simulink model "Virtual_Exhaust_Aftertreatment_Controller_PRT"  (R2016b)
settings: Solver=FixedStepAuto  StartTime=0.0  StopTime=inf  FixedStep=VirtExhATCtrlr.tiSimnTiStep_C  RelTol=1e-3  SampleTimeConstraint=STIndependent  EnableMultiTasking=on
undefined symbols (not defined in the file or in its folder): CAL, SOUIT, T3LIMCL_COEOM_MSK_SY, T3LimCL_stMskEOM1_C, T3LimCL_stMskEOM2_C, T3LimCL_stMskEOM3_C, VirtExhATCtrlr_numHrznSize_CA
libraries: simulink x4
(part 2 of 5)

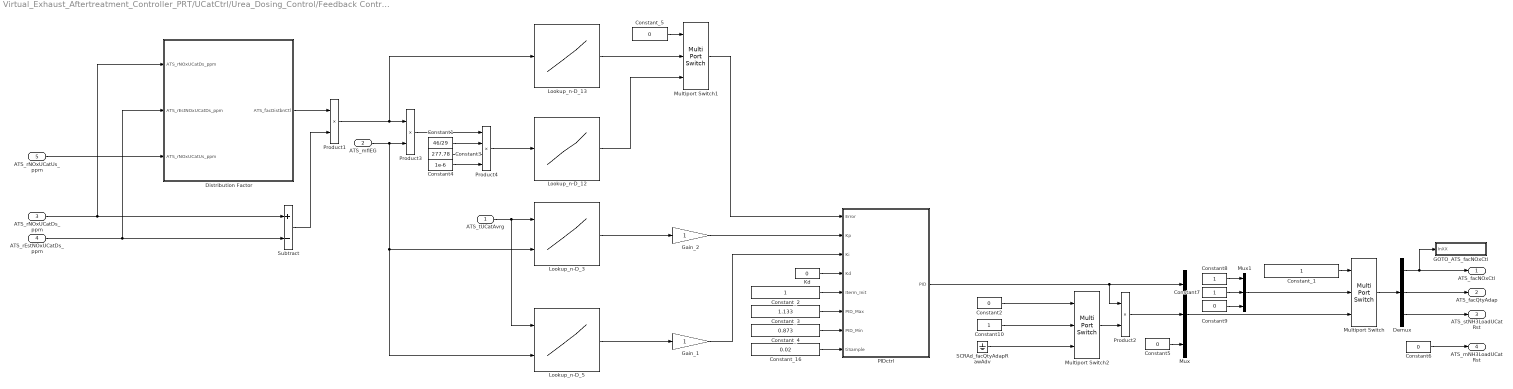
== system Virtual_Exhaust_Aftertreatment_Controller_PRT/UCatCtrl/Urea_Dosing_Control/Feedback Control ==
  "ATS_tUCatAvrg " : Inport
  ATS_mflEG : Inport  Port=2
  "ATS_rNOxUCatDs_ppm " : Inport  Port=3
  ATS_rEstNOxUCatDs_ppm : Inport  Port=4
  ATS_rNOxUCatUs_ppm : Inport  Port=5
  Constant1 : Constant  Value=46/29  SampleTime=-1
  Constant10 : Constant  SampleTime=-1
  Constant{2,5..6,9} (4 alike) : Constant  Value=0  SampleTime=-1
  Constant3 : Constant  Value=277.78  SampleTime=-1
  Constant4 : Constant  Value=1e-6  SampleTime=-1
  Constant7 : Constant  SampleTime=-1
  Constant8 : Constant  SampleTime=-1
  Constant_1 : Constant  SampleTime=-1
  Constant_16 : Constant  Value=0.02  SampleTime=-1
  Constant_2 : Constant  SampleTime=-1
  Constant_3 : Constant  Value=1.133  SampleTime=-1
  Constant_4 : Constant  Value=0.873  SampleTime=-1
  Constant_5 : Constant  Value=0  SampleTime=-1
  Demux : Demux  Outputs=3
  Distribution Factor : Subsystem
  GOTO_ATS_facNOxCtl : Subsystem  mask{SIG='ATS_facNOxCtl'}
      mask prompts: SIG "Log Signal Name"
      mask init: same as Virtual_Exhaust_Aftertreatment_Controller_PRT/UCatCtrl/SCR_Prediction/GOTO_ATS_etaEstNOxCnvUCat
      mask Display: fprintf(SIG);
  Gain_1 : Gain
  Gain_2 : Gain
  Kd : Constant  Value=0  SampleTime=-1
  Lookup_n-D_12 : Lookup_n-D  NumberOfTableDimensions=1  BreakpointsForDimension1=[0;10;20;30;40;50;55;60]  BreakpointsForDimension2=[159.96 449.96]  Table=[1;1;1;1;1;1;1;1]  ExtrapMethod=Clip  UseLastTableValue=on  RndMeth=Simplest  InputSameDT=on
  Lookup_n-D_13 : Lookup_n-D  NumberOfTableDimensions=1  BreakpointsForDimension1=[-500;-300;-50;0;50;100;150;175]  BreakpointsForDimension2=[159.96 449.96]  Table=[-1;-0.5;-0.14;0;0.15;0.4;0.8;1]  ExtrapMethod=Clip  UseLastTableValue=on  RndMeth=Simplest  InputSameDT=on
  Lookup_n-D_3 : Lookup_n-D  BreakpointsForDimension1=[0;200;400;600;800;1000;1200;1400]  BreakpointsForDimension2=[149.96 199.96 249.96 299.96 349.96 399.96 449.96 499.96]  Table=[0.15 0.15 0.15 0.15 0.12 0.09 0.06 0.03;0.136 0.136 0.136 0.136 0.109 0.081 0.054 0.027;0.121 0.121 0.121 0.121 0.097 0.073 0.049 0.024;0.107 0.107 0.107 0.107 0.086 0.064 0.043 0.021;0.093 0.093 0.093 0.093 0.074 0.056 0.037 0.019;0.079 0.079 0.079 0.079 0.063 0.047 0.031 0.016;0.064 0.064 0.064 0.064 0.051 0.039 0.026 0.013;0.05 0.05 0.05 0.05 0.04 0.03 0.02 0.01]  ExtrapMethod=Clip  UseLastTableValue=on  RndMeth=Simplest  InputSameDT=on
  Lookup_n-D_5 : Lookup_n-D  BreakpointsForDimension1=[0;200;400;600;800;1000;1200;1400]  BreakpointsForDimension2=[249.96 299.96 324.96 349.96 374.96 399.96 424.96 449.96]  Table=[0.1 0.068 0.052 0.036 0.02 0.0167 0.0133 0.01;0.1 0.068 0.052 0.036 0.02 0.0167 0.0133 0.01;0.1 0.068 0.052 0.036 0.02 0.0167 0.0133 0.01;0.1 0.068 0.052 0.036 0.02 0.0167 0.0133 0.01;0.1 0.068 0.052 0.036 0.02 0.0167 0.0133 0.01;0.1 0.068 0.052 0.036 0.02 0.0167 0.0133 0.01;0.1 0.068 0.052 0.036 0.02 0.0167 0.0133 0.01;0.1 0.068 0.052 0.036 0.02 0.0167 0.0133 0.01]  ExtrapMethod=Clip  UseLastTableValue=on  RndMeth=Simplest  InputSameDT=on
  Multiport Switch : MultiPortSwitch  DataPortOrder=Zero-based contiguous  Inputs=2
  Multiport Switch1 : MultiPortSwitch  DataPortOrder=Zero-based contiguous  Inputs=2
  Multiport Switch2 : MultiPortSwitch  DataPortOrder=Zero-based contiguous  Inputs=2
  Mux : Mux  Inputs=3
  Mux1 : Mux  Inputs=3
  PIDctrl : Subsystem
  Product1 : Product  RndMeth=Zero
  Product2 : Product  RndMeth=Zero
  Product3 : Product  RndMeth=Zero
  Product4 : Product  Inputs=4  RndMeth=Zero
  SCRAd_facQtyAdapRawAdv : Ground
  Subtract : Sum  Inputs=+-
  ATS_facNOxCtl : Outport
  ATS_facQtyAdap : Outport  Port=2
  ATS_stNH3LoadUCatRst : Outport  Port=3
  ATS_mNH3LoadUCatRst : Outport  Port=4
  wires:
  "ATS_tUCatAvrg "/1 -> Lookup_n-D_5/1, Lookup_n-D_3/1
  Lookup_n-D_5/1 -> Gain_1/1
  ATS_mflEG/1 -> Lookup_n-D_5/2, Lookup_n-D_3/2, Product3/2
  Lookup_n-D_3/1 -> Gain_2/1
  "ATS_rNOxUCatDs_ppm "/1 -> Distribution Factor/1("ATS_rNOxUCatDs_ppm "), Subtract/1
  PIDctrl/1(PID) -> Product2/1, Mux/1
  Subtract/1 -> Product1/2
  Demux/2 -> ATS_facQtyAdap/1
  Multiport Switch2/1 -> Product2/2
  ATS_rEstNOxUCatDs_ppm/1 -> Distribution Factor/2(ATS_rEstNOxUCatDs_ppm), Subtract/2
  ATS_rNOxUCatUs_ppm/1 -> Distribution Factor/3(ATS_rNOxUCatUs_ppm)
  Distribution Factor/1(ATS_facDistbnCtl) -> Product1/1
  Product1/1 -> Lookup_n-D_13/1, Product3/1
  Lookup_n-D_13/1 -> Multiport Switch1/2
  Product3/1 -> Product4/1
  Constant1/1 -> Product4/2
  Constant3/1 -> Product4/3
  Constant4/1 -> Product4/4
  Product4/1 -> Lookup_n-D_12/1
  Constant_5/1 -> Multiport Switch1/1
  Lookup_n-D_12/1 -> Multiport Switch1/3
  Multiport Switch1/1 -> PIDctrl/1(Error)
  Gain_1/1 -> PIDctrl/3(Ki)
  Gain_2/1 -> PIDctrl/2(Kp)
  Constant2/1 -> Multiport Switch2/1
  Constant10/1 -> Multiport Switch2/2
  SCRAd_facQtyAdapRawAdv/1 -> Multiport Switch2/3
  Constant6/1 -> ATS_mNH3LoadUCatRst/1
  Demux/3 -> ATS_stNH3LoadUCatRst/1
  Mux/1 -> Multiport Switch/3
  Constant_1/1 -> Multiport Switch/1
  Mux1/1 -> Multiport Switch/2
  Product2/1 -> Mux/2
  Constant5/1 -> Mux/3
  Constant8/1 -> Mux1/1
  Constant9/1 -> Mux1/3
  Multiport Switch/1 -> Demux/1
  Demux/1 -> ATS_facNOxCtl/1, GOTO_ATS_facNOxCtl/1(InXX)
  Constant_16/1 -> PIDctrl/8(tiSample)
  Kd/1 -> PIDctrl/4(Kd)
  Constant_2/1 -> PIDctrl/5(Iterm_Init)
  Constant_4/1 -> PIDctrl/7(PID_Min)
  Constant7/1 -> Mux1/2
  Constant_3/1 -> PIDctrl/6(PID_Max)

== system Virtual_Exhaust_Aftertreatment_Controller_PRT/UCatCtrl/Urea_Dosing_Control/GOTO_ATS_facQtyAdap ==
  InXX : Inport
  GainXX : Subsystem
  tag scope: ATS_facQtyAdap=global
  wires:
  InXX/1 -> GainXX/1(In)
  GainXX/1(Out) -> [ATS_facQtyAdap]  "ATS_facQtyAdap"

== system Virtual_Exhaust_Aftertreatment_Controller_PRT/UCatCtrl/Urea_Dosing_Control/GOTO_ATS_mNH3LdNom ==
  InXX : Inport
  GainXX : Subsystem
  tag scope: ATS_mNH3LdNom=global
  wires:
  GainXX/1(Out) -> [ATS_mNH3LdNom]  "ATS_mNH3LdNom"
  InXX/1 -> GainXX/1(In)

== system Virtual_Exhaust_Aftertreatment_Controller_PRT/UCatCtrl/Urea_Dosing_Control/GOTO_ATS_mNH3LoadUCatRst ==
  InXX : Inport
  GainXX : Subsystem
  tag scope: ATS_mNH3LoadUCatRst=global
  wires:
  InXX/1 -> GainXX/1(In)
  GainXX/1(Out) -> [ATS_mNH3LoadUCatRst]  "ATS_mNH3LoadUCatRst"

== system Virtual_Exhaust_Aftertreatment_Controller_PRT/UCatCtrl/Urea_Dosing_Control/GOTO_ATS_mflNH3Cnv_mgps ==
  InXX : Inport
  GainXX : Subsystem
  tag scope: ATS_mflNH3Cnv_mgps=global
  wires:
  InXX/1 -> GainXX/1(In)
  GainXX/1(Out) -> [ATS_mflNH3Cnv_mgps]  "ATS_mflNH3Cnv_mgps"

== system Virtual_Exhaust_Aftertreatment_Controller_PRT/UCatCtrl/Urea_Dosing_Control/GOTO_ATS_mflNH3CurrEfc_mgps ==
  InXX : Inport
  GainXX : Subsystem
  tag scope: ATS_mflNH3CurrEfc_mgps=global
  wires:
  InXX/1 -> GainXX/1(In)
  GainXX/1(Out) -> [ATS_mflNH3CurrEfc_mgps]  "ATS_mflNH3CurrEfc_mgps"

== system Virtual_Exhaust_Aftertreatment_Controller_PRT/UCatCtrl/Urea_Dosing_Control/GOTO_ATS_mflNH3DpstLmt_mgps ==
  InXX : Inport
  GainXX : Subsystem
  tag scope: ATS_mflNH3DpstLmt_mgps=global
  wires:
  GainXX/1(Out) -> [ATS_mflNH3DpstLmt_mgps]  "ATS_mflNH3DpstLmt_mgps"
  InXX/1 -> GainXX/1(In)

== system Virtual_Exhaust_Aftertreatment_Controller_PRT/UCatCtrl/Urea_Dosing_Control/GOTO_ATS_mflNH3MetAdapDes_mgps ==
  InXX : Inport
  GainXX : Subsystem
  tag scope: ATS_mflNH3MetAdapDes_mgps=global
  wires:
  GainXX/1(Out) -> [ATS_mflNH3MetAdapDes_mgps]  "ATS_mflNH3MetAdapDes_mgps"
  InXX/1 -> GainXX/1(In)

== system Virtual_Exhaust_Aftertreatment_Controller_PRT/UCatCtrl/Urea_Dosing_Control/GOTO_ATS_mflNH3PreCtl_mgps ==
  InXX : Inport
  GainXX : Subsystem
  tag scope: ATS_mflNH3PreCtl_mgps=global
  wires:
  InXX/1 -> GainXX/1(In)
  GainXX/1(Out) -> [ATS_mflNH3PreCtl_mgps]  "ATS_mflNH3PreCtl_mgps"

== system Virtual_Exhaust_Aftertreatment_Controller_PRT/UCatCtrl/Urea_Dosing_Control/GOTO_ATS_mflNH3_mgps ==
  InXX : Inport
  GainXX : Subsystem
  tag scope: ATS_mflNH3_mgps=global
  wires:
  InXX/1 -> GainXX/1(In)
  GainXX/1(Out) -> [ATS_mflNH3_mgps]  "ATS_mflNH3_mgps"

== system Virtual_Exhaust_Aftertreatment_Controller_PRT/UCatCtrl/Urea_Dosing_Control/GOTO_ATS_mflNOxUs_mgps ==
  InXX : Inport
  GainXX : Subsystem
  tag scope: ATS_mflNOxUs_mgps=global
  wires:
  GainXX/1(Out) -> [ATS_mflNOxUs_mgps]  "ATS_mflNOxUs_mgps"
  InXX/1 -> GainXX/1(In)

== system Virtual_Exhaust_Aftertreatment_Controller_PRT/UCatCtrl/Urea_Dosing_Control/GOTO_ATS_stNH3LoadUCatRst ==
  InXX : Inport
  GainXX : Subsystem
  tag scope: ATS_stNH3LoadUCatRst=global
  wires:
  GainXX/1(Out) -> [ATS_stNH3LoadUCatRst]  "ATS_stNH3LoadUCatRst"
  InXX/1 -> GainXX/1(In)

== system Virtual_Exhaust_Aftertreatment_Controller_PRT/UCatCtrl/Urea_Dosing_Control/GOTO_ATS_stUDosing ==
  InXX : Inport
  GainXX : Subsystem
  tag scope: ATS_stUDosing=global
  wires:
  InXX/1 -> GainXX/1(In)
  GainXX/1(Out) -> [ATS_stUDosing]  "ATS_stUDosing"

== system Virtual_Exhaust_Aftertreatment_Controller_PRT/UCatCtrl/Urea_Dosing_Control/GOTO_EvpMod_tUCatUsT ==
  InXX : Inport
  GainXX : Subsystem
  tag scope: EvpMod_tUCatUsT=global
  wires:
  InXX/1 -> GainXX/1(In)
  GainXX/1(Out) -> [EvpMod_tUCatUsT]  "EvpMod_tUCatUsT"

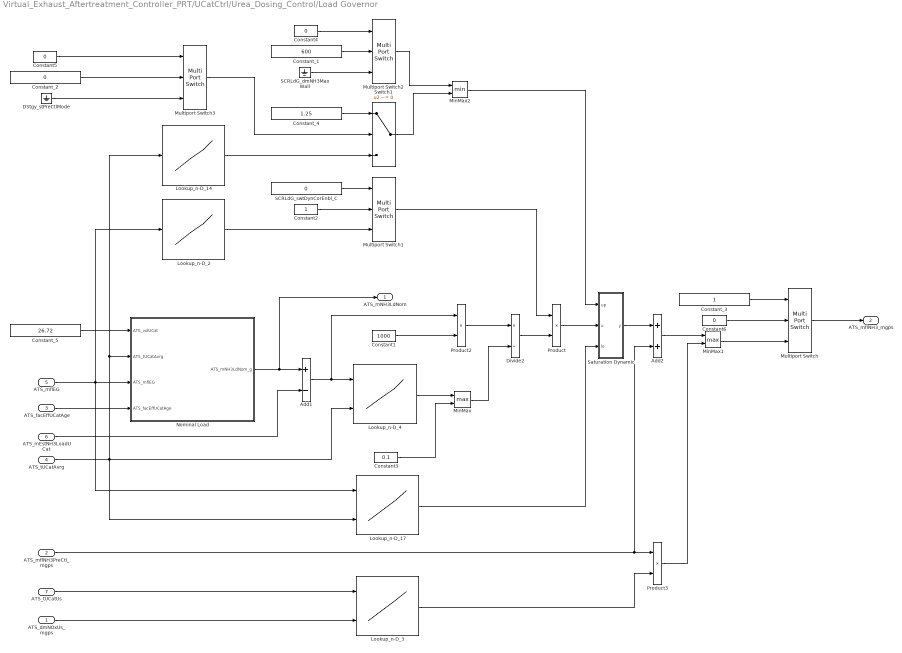
== system Virtual_Exhaust_Aftertreatment_Controller_PRT/UCatCtrl/Urea_Dosing_Control/Load Governor ==
  ATS_dmNOxUs_mgps : Inport
  ATS_mflNH3PreCtl_mgps : Inport  Port=2
  ATS_facEffUCatAge : Inport  Port=3
  ATS_tUCatAvrg : Inport  Port=4
  ATS_mflEG : Inport  Port=5
  ATS_mEstNH3LoadUCat : Inport  Port=6
  ATS_tUCatUs : Inport  Port=7
  Add1 : Sum  Inputs=+-
  Add2 : Sum
  Constant1 : Constant  Value=1000  SampleTime=-1
  Constant2 : Constant  SampleTime=-1
  Constant3 : Constant  Value=0.1  SampleTime=-1
  Constant4 : Constant  Value=0  SampleTime=-1
  Constant5 : Constant  Value=0  SampleTime=-1
  Constant6 : Constant  Value=0  SampleTime=-1
  Constant_1 : Constant  Value=600  SampleTime=-1
  Constant_2 : Constant  Value=0  SampleTime=-1
  Constant_3 : Constant  SampleTime=-1
  Constant_4 : Constant  Value=1.25  SampleTime=-1
  Constant_5 : Constant  Value=26.72  SampleTime=-1
  DStgy_stPreCtlMode : Ground
  Divide2 : Product  Inputs=*/
  Lookup_n-D_14 : Lookup_n-D  NumberOfTableDimensions=1  BreakpointsForDimension1=[159.96;229.96;299.96;369.96;439.96;509.96;579.96;649.96]  BreakpointsForDimension2=[159.96 449.96]  Table=[365;365;365;365;365;365;365;365]  ExtrapMethod=Clip  UseLastTableValue=on  RndMeth=Simplest  InputSameDT=on
  Lookup_n-D_17 : Lookup_n-D  BreakpointsForDimension1=[100;300;500;700;900;1100;1300;1500;1700;1900]  BreakpointsForDimension2=[159.96 449.96]  Table=[-50 -70;-55 -80;-65 -90;-75 -100;-90 -120;-105 -150;-130 -180;-160 -220;-195 -290;-250 -365]  ExtrapMethod=Clip  UseLastTableValue=on  RndMeth=Simplest  InputSameDT=on
  Lookup_n-D_2 : Lookup_n-D  NumberOfTableDimensions=1  BreakpointsForDimension1=[150;250;350;500;700;1000;1250;1500]  BreakpointsForDimension2=[159.96 449.96]  Table=[1;1;1;1;1;0.98;0.95;0.92]  ExtrapMethod=Clip  UseLastTableValue=on  RndMeth=Simplest  InputSameDT=on
  Lookup_n-D_3 : Lookup_n-D  BreakpointsForDimension1=[99.96;199.96;299.96;399.96;499.96;599.96]  BreakpointsForDimension2=[0 100 200 300 400 500]  Table=[0.5 0.5 0.5 0.5 0.5 0.5;0.5 0.5 0.5 0.5 0.5 0.5;0.5 0.5 0.5 0.5 0.5 0.5;0.5 0.5 0.5 0.5 0.5 0.5;0.5 0.5 0.5 0.5 0.5 0.5;0.5 0.5 0.5 0.5 0.5 0.5]  ExtrapMethod=Clip  UseLastTableValue=on  RndMeth=Simplest  InputSameDT=on
  Lookup_n-D_4 : Lookup_n-D  BreakpointsForDimension1=[-10;-5;-3;-2;-1;0.025000000372529;1;2;3;5;10]  BreakpointsForDimension2=[159.96 449.96]  Table=[27.5 27.5;43 35;57 45;65 60;74 74;70 0.1;35 2.8;25 5.5;22 8.3;22 13.8;27.5 27.5]  ExtrapMethod=Clip  UseLastTableValue=on  RndMeth=Simplest  InputSameDT=on
  MinMax : MinMax  Function=max  Inputs=2
  MinMax1 : MinMax  Function=max  Inputs=2
  MinMax2 : MinMax  Inputs=2
  Multiport Switch{,1..3} (4 alike) : MultiPortSwitch  DataPortOrder=Zero-based contiguous  Inputs=2
  Nominal Load : Subsystem
  Product : Product
  Product2 : Product  RndMeth=Zero
  Product3 : Product
  SCRLdG_dmNH3MaxWall : Ground
  SCRLdG_swtDynCorEnbl_C : Constant  Value=0  SampleTime=-1
  Saturation Dynamic : Subsystem  mask(Saturation Dynamic){OutMin=[], OutMax=[], OutDataTypeStr=Inherit: Same as second input, OutputDataTypeScalingMode=Same as second input, OutDataType=fixdt(1, 16), OutScaling=2^-10, LockScale=off, RndMeth=Floor, DoSatur=off}
      mask prompts: OutMin "Simulink:masks:OutputMinimum_MP"; OutMax "Simulink:masks:OutputMaximum_MP"; OutDataTypeStr "Simulink:masks:OutputDataType_MP"; OutputDataTypeScalingMode "Simulink:masks:OutputDataTypeMode_MP"; OutDataType "Simulink:masks:OutputDataTypeegFixdt116Fixdtsingle_MP"; OutScaling "Simulink:masks:OutputScalingSlopeEg29OrSlopeBias_MP"; LockScale "Simulink:masks:LockOutputDataTypeAgainstFxpTools_MP"; RndMeth "Simulink:masks:IntegerRoundingMode_MP"; DoSatur "Simulink:masks:SaturateOnIntegerOverflow_MP"
      mask help: Simulink:masks:SaturationDynamic_MD
      mask init: same as Virtual_Exhaust_Aftertreatment_Controller_PRT/UCatCtrl/Urea_Dosing_Control/Saturation Dynamic
      mask Callback OutDataTypeStr: fixptdialog(gcbh)
      mask TypeOptions OutputDataTypeScalingMode: double | single | int8 | uint8 | int16 | uint16 | int32 | uint32 | Specify via dialog | Same as second input
      mask Callback OutputDataTypeScalingMode: fixptdialog(gcbh)
      mask Callback OutDataType: fixptdialog(gcbh)
      mask TypeOptions RndMeth: Simulink:masks:Ceiling | Simulink:masks:Convergent | Simulink:masks:Floor | Simulink:masks:Nearest | Simulink:masks:Round | Simulink:masks:Simplest | Simulink:masks:Zero
      mask Display: plot([0.15 0.85],[.5 .5],[.5 .5],[0.05 0.95],0.15+0.7*[0 .25 .75 1],0.05+0.9*[.25 .25 .75 .75]);
  Switch1 : Switch  Criteria=u2 ~= 0  Threshold=SOUIT
  ATS_mNH3LdNom : Outport
  ATS_mflNH3_mgps : Outport  Port=2
  wires:
  Nominal Load/1(ATS_mNH3LdNom_g) -> ATS_mNH3LdNom/1, Add1/1
  ATS_mEstNH3LoadUCat/1 -> Add1/2
  Add1/1 -> Lookup_n-D_4/1, Product2/1
  ATS_tUCatAvrg/1 -> Nominal Load/2(ATS_tUCatAvrg), Lookup_n-D_14/1, Lookup_n-D_17/2, Lookup_n-D_4/2
  Lookup_n-D_4/1 -> MinMax/1
  Constant3/1 -> MinMax/2
  Constant1/1 -> Product2/2
  Product2/1 -> Divide2/1
  MinMax/1 -> Divide2/2
  ATS_mflNH3PreCtl_mgps/1 -> Add2/2, Product3/1
  MinMax1/1 -> Multiport Switch/3
  ATS_facEffUCatAge/1 -> Nominal Load/4(ATS_facEffUCatAge)
  Constant_5/1 -> Nominal Load/1(ATS_volUCat)
  Lookup_n-D_17/1 -> Saturation Dynamic/3(lo)
  Saturation Dynamic/1(y) -> Add2/1
  Product/1 -> Saturation Dynamic/2(u)
  Lookup_n-D_2/1 -> Multiport Switch1/3
  ATS_mflEG/1 -> Lookup_n-D_2/1, Lookup_n-D_17/1, Nominal Load/3(ATS_mflEG)
  Lookup_n-D_3/1 -> Product3/2
  Product3/1 -> MinMax1/2
  Divide2/1 -> Product/2
  Add2/1 -> MinMax1/1
  SCRLdG_swtDynCorEnbl_C/1 -> Multiport Switch1/1
  Constant2/1 -> Multiport Switch1/2
  Multiport Switch1/1 -> Product/1
  Lookup_n-D_14/1 -> Switch1/3
  Switch1/1 -> MinMax2/2
  Multiport Switch2/1 -> MinMax2/1
  MinMax2/1 -> Saturation Dynamic/1(up)
  ATS_tUCatUs/1 -> Lookup_n-D_3/1
  ATS_dmNOxUs_mgps/1 -> Lookup_n-D_3/2
  SCRLdG_dmNH3MaxWall/1 -> Multiport Switch2/3
  Constant4/1 -> Multiport Switch2/1
  Constant_1/1 -> Multiport Switch2/2
  Constant_4/1 -> Switch1/1
  Constant5/1 -> Multiport Switch3/1
  DStgy_stPreCtlMode/1 -> Multiport Switch3/3
  Constant_2/1 -> Multiport Switch3/2
  Multiport Switch3/1 -> Switch1/2
  Constant_3/1 -> Multiport Switch/1
  Constant6/1 -> Multiport Switch/2
  Multiport Switch/1 -> ATS_mflNH3_mgps/1

== system Virtual_Exhaust_Aftertreatment_Controller_PRT/UCatCtrl/Urea_Dosing_Control/SCRMod Wall Film ==
  ATS_mflNH3Cnv_mgps : Inport
  Constant_1 : Constant  Value=0  SampleTime=-1
  Multiport Switch1 : MultiPortSwitch  DataPortOrder=Zero-based contiguous  Inputs=2
  SCRMod_dmNH3CurrEff : Ground
  ATS_mflNH3CurrEfc_mgps : Outport
  wires:
  SCRMod_dmNH3CurrEff/1 -> Multiport Switch1/3
  Constant_1/1 -> Multiport Switch1/1
  Multiport Switch1/1 -> ATS_mflNH3CurrEfc_mgps/1
  ATS_mflNH3Cnv_mgps/1 -> Multiport Switch1/2

== system Virtual_Exhaust_Aftertreatment_Controller_PRT/UCatCtrl/Urea_Dosing_Control/Saturation Dynamic ==
  up : Inport
  u : Inport  Port=2
  lo : Inport  Port=3
  Data Type Duplicate : DataTypeDuplicate  DisableCoverage=on
  Data Type Propagation : S-Function  FunctionName=sfix_dtprop  Parameters=14,PropDataTypeMode,(getdatatypespecs(PropDataType,PropScaling,DblOver,0, 0, PropDataTypeMode, PropScalingMode)),IfRefDouble,IfRefSingle,IsSigned,NumBitsBase,NumBitsMult,NumBitsAdd,(sort(reshape(round(NumBitsAllowFinal), prod(size(NumBitsAllowFinal)),1))),PropScalingMode,ValuesUsedBestPrec,SlopeBase,SlopeMult,SlopeAdd,BiasBase,BiasMult,BiasAdd,DblOver  SFunctionDeploymentMode=off  EnableBusSupport=off  mask(Data Type Propagation){PropDataTypeMode=Inherit via propagation rule, PropDataType=fixdt(1, 16), IfRefDouble=double, IfRefSingle=single, IsSigned=IsSigned1, NumBitsBase=NumBits1, NumBitsMult=1, NumBitsAdd=0, NumBitsAllowFinal=1:128, PropScalingMode=Inherit via propagation rule, PropScaling=2^-10, ValuesUsedBestPrec=[5 -7], SlopeBase=Slope1, SlopeMult=1, SlopeAdd=0, BiasBase=Bias1, BiasMult=1, BiasAdd=0}
      mask prompts: PropDataTypeMode "Simulink:masks:x1PropagatedDataType_MP"; PropDataType "Simulink:masks:x11PropagatedDataTypeegFixdt116Fixdtsingle_MP"; IfRefDouble "Simulink:masks:x11IfAnyReferenceInputIsDoubleOutputIs_MP"; IfRefSingle "Simulink:masks:x12IfAnyReferenceInputIsSingleOutputIs_MP"; IsSigned "Simulink:masks:x13IsSigned_MP"; NumBitsBase "Simulink:masks:x141NumberofBitsBase_MP"; NumBitsMult "Simulink:masks:x142NumberofBitsMultiplicativeAdjustment_MP"; NumBitsAdd "Simulink:masks:x143NumberofBitsAdditiveAdjustment_MP"; NumBitsAllowFinal "Simulink:masks:x144NumberofBitsAllowableFinalValues_MP"; PropScalingMode "Simulink:masks:x2PropagatedScaling_MP"; PropScaling "Simulink:masks:x21PropagatedScalingSlopeEg29OrSlopeBiasEg1253_MP"; ValuesUsedBestPrec "Simulink:masks:x21ValuesUsedToDetermineBestPrecisionScaling_MP"; SlopeBase "Simulink:masks:x211SlopeBase_MP"; SlopeMult "Simulink:masks:x212SlopeMultiplicativeAdjustment_MP"; SlopeAdd "Simulink:masks:x213SlopeAdditiveAdjustment_MP"; BiasBase "Simulink:masks:x221BiasBase_MP"; BiasMult "Simulink:masks:x222BiasMultiplicativeAdjustment_MP"; BiasAdd "Simulink:masks:x223BiasAdditiveAdjustment_MP"
      mask help: Simulink:masks:DataTypePropagation_MD
      mask init:
      | DblOver = 0;
      mask TypeOptions PropDataTypeMode: Simulink:masks:SpecifyViaDialog | Simulink:masks:InheritViaPropagationRule
      mask Callback PropDataTypeMode: fixptdialog(gcbh)
      mask Callback PropDataType: fixptdialog(gcbh)
      mask TypeOptions IfRefDouble: Simulink:masks:double | Simulink:masks:single
      mask TypeOptions IfRefSingle: Simulink:masks:double | Simulink:masks:single
      mask TypeOptions IsSigned: Simulink:masks:IsSigned1 | Simulink:masks:IsSigned2 | Simulink:masks:IsSigned1OrIsSigned2 | Simulink:masks:TRUE | Simulink:masks:FALSE
      mask TypeOptions NumBitsBase: NumBits1 | NumBits2 | max([NumBits1 NumBits2]) | min([NumBits1 NumBits2]) | NumBits1+NumBits2
      mask TypeOptions PropScalingMode: Simulink:masks:SpecifyViaDialog | Simulink:masks:InheritViaPropagationRule | Simulink:masks:ObtainViaBestPrecision
      mask Callback PropScalingMode: fixptdialog(gcbh)
      mask TypeOptions SlopeBase: Slope1 | Slope2 | max([Slope1 Slope2]) | min([Slope1 Slope2]) | Slope1*Slope2 | Slope1/Slope2 | PosRange1 | PosRange2 | max([PosRange1 PosRange2]) | min([PosRange1 PosRange2]) | PosRange1*PosRange2 | PosRange1/PosRange2
      mask TypeOptions BiasBase: Bias1 | Bias2 | max([Bias1 Bias2]) | min([Bias1 Bias2]) | Bias1*Bias2 | Bias1/Bias2 | Bias1+Bias2 | Bias1-Bias2
      mask Display:
      | port_label('Input',1,'Ref1');
      | port_label('Input',2,'Ref2');
      | port_label('Input',3,'Prop');
  LowerRelop1 : RelationalOperator  DisableCoverage=on  Operator=>  OutDataTypeStr=boolean  RndMeth=Nearest
  Switch : Switch  Criteria=u2 ~= 0  OutDataTypeStr=Inherit: Inherit via back propagation  ZeroCross=off
  Switch2 : Switch  Criteria=u2 ~= 0  OutMin=OutMin  OutMax=OutMax  OutDataTypeStr=Inherit: Inherit via back propagation  ZeroCross=off
  UpperRelop : RelationalOperator  DisableCoverage=on  Operator=<  OutDataTypeStr=boolean  RndMeth=Nearest
  y : Outport  OutMin=OutMin  OutMax=OutMax
  wires:
  up/1 -> Switch2/1, LowerRelop1/2
  u/1 -> Data Type Propagation/2, Data Type Propagation/1, LowerRelop1/1, Switch/3, UpperRelop/1
  lo/1 -> Switch/1, UpperRelop/2
  Switch/1 -> Data Type Duplicate/2, Switch2/3, Data Type Propagation/3
  Switch2/1 -> Data Type Duplicate/1, y/1
  LowerRelop1/1 -> Switch2/2
  UpperRelop/1 -> Switch/2

== system Virtual_Exhaust_Aftertreatment_Controller_PRT/UCatCtrl/SCR_Prediction/GOTO_ATS_etaEstNOxCnvUCat/GainXX ==
  In : Inport
  Out : Outport
  wires:
  In/1 -> Out/1

== system Virtual_Exhaust_Aftertreatment_Controller_PRT/UCatCtrl/SCR_Prediction/GOTO_ATS_facEstEfcUCatAge/GainXX ==
  In : Inport
  Out : Outport
  wires:
  In/1 -> Out/1

== system Virtual_Exhaust_Aftertreatment_Controller_PRT/UCatCtrl/SCR_Prediction/GOTO_ATS_mEstNH3LoadUCat/GainXX ==
  In : Inport
  Out : Outport
  wires:
  In/1 -> Out/1

== system Virtual_Exhaust_Aftertreatment_Controller_PRT/UCatCtrl/SCR_Prediction/GOTO_ATS_mflEstNH3OxiUCatUs_mgps/GainXX ==
  In : Inport
  Out : Outport
  wires:
  In/1 -> Out/1

== system Virtual_Exhaust_Aftertreatment_Controller_PRT/UCatCtrl/SCR_Prediction/GOTO_ATS_rEstNOxUCatDs_ppm/GainXX ==
  In : Inport
  Out : Outport
  wires:
  In/1 -> Out/1

== system Virtual_Exhaust_Aftertreatment_Controller_PRT/UCatCtrl/SCR_Prediction/GOTO_ATS_tEstUCatAvrg/GainXX ==
  In : Inport
  Out : Outport
  wires:
  In/1 -> Out/1

== system Virtual_Exhaust_Aftertreatment_Controller_PRT/UCatCtrl/SCR_Prediction/Main/Aging Prediction ==
  ATS_tAvrg : Inport
  Constant5 : Constant  SampleTime=-1
  Ground_ATS_GlbDa_ITotDst : Ground
  Terminator : Terminator
  estAging : Subsystem  Commented=on
  ATS_facEstEfcUCatAge : Outport
  wires:
  Constant5/1 -> ATS_facEstEfcUCatAge/1
  Ground_ATS_GlbDa_ITotDst/1 -> estAging/2(ATS_GlbDa_ITotDst)
  ATS_tAvrg/1 -> estAging/1(ATS_tAvrg)
  estAging/1(ATS_facEstEfcUCatAge) -> Terminator/1

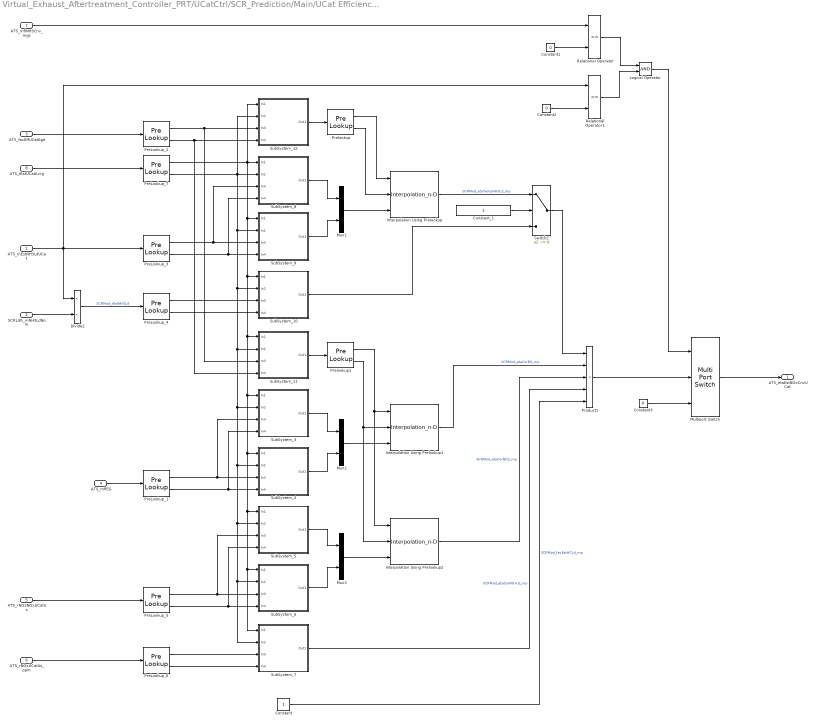
== system Virtual_Exhaust_Aftertreatment_Controller_PRT/UCatCtrl/SCR_Prediction/Main/UCat Efficiency Prediction ==
  ATS_mEstNH3LdUCat : Inport
  SCRLdG_mNH3LdNom : Inport  Port=2
  ATS_facEffUCatAge : Inport  Port=3
  ATS_mflEG : Inport  Port=4
  ATS_rNO2NOxUCatUs : Inport  Port=5
  ATS_rNOxUCatUs_ppm : Inport  Port=6
  ATS_mflNH3Cnv_mgs : Inport  Port=7
  ATS_tEstUCatAvrg : Inport  Port=8
  Constant : Constant  SampleTime=-1
  Constant1 : Constant  Value=0  SampleTime=-1
  Constant2 : Constant  Value=0  SampleTime=-1
  Constant3 : Constant  Value=0  SampleTime=-1
  Constant_1 : Constant  SampleTime=-1
  Divide2 : Product  Inputs=*/
  Interpolation Using Prelookup : Interpolation_n-D  NumberOfTableDimensions=1  TableSource=Input port  Table=|  ExtrapMethod=Clip  ValidIndexMayReachLast=on
      | [    0.2790    0.2970    0.3080    0.3220    0.3510    0.4240    0.5640    0.6550    0.8190    1.0000    1.0000    1.0000
      |     0.3260    0.3430    0.3540    0.3670    0.3960    0.4660    0.6010    0.6900    0.8440    1.0000    1.0000    1.0000
      |     0.3730    0.3890    0.4000    0.4130    0.4400    0.5080    0.6380    0.7230    0.8680    1.0000    1.0000    1.0000
      |     0.4320    0.4480    0.4580    0.4700    0.4960    0.5600    0.6830    0.7640    0.8970    1.0000    1.0000    1.0000
      |     0.4920    0.5070    0.5160    0.5270    0.5520    0.6120    0.7260    0.8020    0.9220    1.0000    1.0000    1.0000
      |     0.5510    0.5650    0.5730    0.5840    0.6070    0.6620    0.7680    0.8370    0.9410    1.0000    1.0000    1.0000
      |     0.6070    0.6200    0.6280    0.6380    0.6600    0.7130    0.8130    0.8750    0.9580    1.0000    1.0000    1.0000
      |     0.6580    0.6710    0.6790    0.6890    0.7110    0.7630    0.8600    0.9130    0.9730    1.0000    1.0000    1.0000
      |     0.7030    0.7170    0.7250    0.7360    0.7580    0.8130    0.9110    0.9540    0.9900    1.0000    1.0000    1.0000
      |     0.7620    0.7790    0.7900    0.8030    0.8300    0.8980    1.0000    1.0000    1.0000    1.0000    1.0000    1.0000
      |     0.7840    0.7980    0.8060    0.8160    0.8370    0.8910    0.9920    1.0000    1.0000    1.0000    1.0000    1.0000
      |     0.7800    0.8780    0.8820    0.8860    0.8950    0.9180    0.9620    1.0000    1.0000    1.0000    1.0000    1.0000
      | ]
      settings: InputPortMap=u0,u1,p2
  Interpolation Using Prelookup1 : Interpolation_n-D  NumberOfTableDimensions=1  TableSource=Input port  Table=|  ExtrapMethod=Clip  ValidIndexMayReachLast=on
      | [    0.2790    0.2970    0.3080    0.3220    0.3510    0.4240    0.5640    0.6550    0.8190    1.0000    1.0000    1.0000
      |     0.3260    0.3430    0.3540    0.3670    0.3960    0.4660    0.6010    0.6900    0.8440    1.0000    1.0000    1.0000
      |     0.3730    0.3890    0.4000    0.4130    0.4400    0.5080    0.6380    0.7230    0.8680    1.0000    1.0000    1.0000
      |     0.4320    0.4480    0.4580    0.4700    0.4960    0.5600    0.6830    0.7640    0.8970    1.0000    1.0000    1.0000
      |     0.4920    0.5070    0.5160    0.5270    0.5520    0.6120    0.7260    0.8020    0.9220    1.0000    1.0000    1.0000
      |     0.5510    0.5650    0.5730    0.5840    0.6070    0.6620    0.7680    0.8370    0.9410    1.0000    1.0000    1.0000
      |     0.6070    0.6200    0.6280    0.6380    0.6600    0.7130    0.8130    0.8750    0.9580    1.0000    1.0000    1.0000
      |     0.6580    0.6710    0.6790    0.6890    0.7110    0.7630    0.8600    0.9130    0.9730    1.0000    1.0000    1.0000
      |     0.7030    0.7170    0.7250    0.7360    0.7580    0.8130    0.9110    0.9540    0.9900    1.0000    1.0000    1.0000
      |     0.7620    0.7790    0.7900    0.8030    0.8300    0.8980    1.0000    1.0000    1.0000    1.0000    1.0000    1.0000
      |     0.7840    0.7980    0.8060    0.8160    0.8370    0.8910    0.9920    1.0000    1.0000    1.0000    1.0000    1.0000
      |     0.7800    0.8780    0.8820    0.8860    0.8950    0.9180    0.9620    1.0000    1.0000    1.0000    1.0000    1.0000
      | ]
      settings: InputPortMap=u0,u1,p2
  Interpolation Using Prelookup2 : Interpolation_n-D  NumberOfTableDimensions=1  TableSource=Input port  Table=|  ExtrapMethod=Clip  ValidIndexMayReachLast=on
      | [    0.2790    0.2970    0.3080    0.3220    0.3510    0.4240    0.5640    0.6550    0.8190    1.0000    1.0000    1.0000
      |     0.3260    0.3430    0.3540    0.3670    0.3960    0.4660    0.6010    0.6900    0.8440    1.0000    1.0000    1.0000
      |     0.3730    0.3890    0.4000    0.4130    0.4400    0.5080    0.6380    0.7230    0.8680    1.0000    1.0000    1.0000
      |     0.4320    0.4480    0.4580    0.4700    0.4960    0.5600    0.6830    0.7640    0.8970    1.0000    1.0000    1.0000
      |     0.4920    0.5070    0.5160    0.5270    0.5520    0.6120    0.7260    0.8020    0.9220    1.0000    1.0000    1.0000
      |     0.5510    0.5650    0.5730    0.5840    0.6070    0.6620    0.7680    0.8370    0.9410    1.0000    1.0000    1.0000
      |     0.6070    0.6200    0.6280    0.6380    0.6600    0.7130    0.8130    0.8750    0.9580    1.0000    1.0000    1.0000
      |     0.6580    0.6710    0.6790    0.6890    0.7110    0.7630    0.8600    0.9130    0.9730    1.0000    1.0000    1.0000
      |     0.7030    0.7170    0.7250    0.7360    0.7580    0.8130    0.9110    0.9540    0.9900    1.0000    1.0000    1.0000
      |     0.7620    0.7790    0.7900    0.8030    0.8300    0.8980    1.0000    1.0000    1.0000    1.0000    1.0000    1.0000
      |     0.7840    0.7980    0.8060    0.8160    0.8370    0.8910    0.9920    1.0000    1.0000    1.0000    1.0000    1.0000
      |     0.7800    0.8780    0.8820    0.8860    0.8950    0.9180    0.9620    1.0000    1.0000    1.0000    1.0000    1.0000
      | ]
      settings: InputPortMap=u0,u1,p2
  Logical Operator : Logic  AllPortsSameDT=off  OutDataTypeStr=boolean
  Multiport Switch : MultiPortSwitch  DataPortOrder=Zero-based contiguous  Inputs=2
  Mux1 : Mux  Inputs=2
  Mux2 : Mux  Inputs=2
  Mux3 : Mux  Inputs=2
  PreLookup_1 : PreLookup  BreakpointsData=[0;100;200;300;400;500;600;700;800;900;1000;1500]  UseLastBreakpoint=on
  PreLookup_2 : PreLookup  BreakpointsData=[0;0.1;0.2;0.3;0.4;0.5;0.6;1]  UseLastBreakpoint=on
  PreLookup_3 : PreLookup  BreakpointsData=[0;0.24;0.38;0.55;0.92;1.85;3.66;4.81;7.39;9.62;24.05;34.2]  UseLastBreakpoint=on
  PreLookup_4 : PreLookup  BreakpointsData=[0;0.1;0.2;0.3;0.4;0.5;0.6;0.7;0.8;0.9;0.95;1]  UseLastBreakpoint=on
  PreLookup_5 : PreLookup  BreakpointsData=[0;0.1;0.2;0.3;0.4;0.5;0.6;0.7;0.8;0.9;0.99;1]  UseLastBreakpoint=on
  PreLookup_6 : PreLookup  BreakpointsData=[0;125;250;500;750;1000;1200;1400;1600;1800;2000;2500]  UseLastBreakpoint=on
  PreLookup_7 : PreLookup  BreakpointsData=[159.96;179.96;199.96;224.96;249.96;274.96;299.96;324.96;349.96;399.96;449.96;599.96]  UseLastBreakpoint=on
  Prelookup : PreLookup  BreakpointsData=|  UseLastBreakpoint=on
      | [  0 1.0
      | ]
  Prelookup1 : PreLookup  BreakpointsData=|  UseLastBreakpoint=on
      | [  0 1.0
      | ]
  Product1 : Product  Inputs=5  RndMeth=Zero
  Relational Operator : RelationalOperator  Operator===  OutDataTypeStr=boolean  RndMeth=Nearest
  Relational Operator1 : RelationalOperator  Operator===  OutDataTypeStr=boolean  RndMeth=Nearest
  SubSystem_10 : Subsystem  mask{table=[1 1 1 1 1 1 1 1 1 1 1 1;1 1 1 1 1 1 1 1 1 1 1 1;1 1 1 1 1 1 1 1 1 1 1 1;1 1 1 1 1 1 1 1 1 1 1 1;1 1 1 1 1 1 1 1 1 1 1 1;1 1 1 1 1 1 1 1 1 1 1 1;1 1 1 1 1 1 1 1 1 1 1 1;1 1 1 1 1 1 1 1 1 1 1 1;1 1 1 1 1 1 1 1 1 1 1 1;1 1 1 1 1 1 1 1 1 1 1 1;1 1 1 1 1 1 1 1 1 1 1 1;1 1 1 1 1 1 1 1 1 1 1 1], row_idx=[159.96;179.96;199.96;224.96;249.96;274.96;299.96;324.96;349.96;399.96;449.96;599.96], col_idx=[0 0.1 0.2 0.3 0.4 0.5 0.6 0.7 0.8 0.9 0.95 1]}
      mask prompts: table "Table Data"; row_idx "Breakpoints 1:"; col_idx "Breakpoints 2:"
      mask Display:
      | color('red');
      | fprintf('Prelookup\n2D');
      | 
      | color('black');
      | port_label('input', 1, 'u1');
      | port_label('input', 2, 'u2');
      | port_label('input', 3, 'u3');
      | port_label('input', 4, 'u4');
  SubSystem_11 : Subsystem  mask{table=[0 0.1 0.2 0.3 0.4 0.5 0.6 1;0 0.1 0.2 0.3 0.4 0.5 0.6 1;0 0.1 0.2 0.3 0.4 0.5 0.6 1;0 0.1 0.2 0.3 0.4 0.5 0.6 1;0 0.1 0.2 0.3 0.4 0.5 0.6 1;0 0.1 0.2 0.3 0.4 0.5 0.6 1;0 0.1 0.2 0.3 0.4 0.5 0.6 1;0 0.1 0.2 0.3 0.4 0.5 0.6 1;0 0.1 0.2 0.3 0.4 0.5 0.6 1;0 0.1 0.2 0.3 0.4 0.5 0.6 1;0 0.1 0.2 0.3 0.4 0.5 0.6 1;0 0.1 0.2 0.3 0.4 0.5 0.6 1], row_idx=[159.96;179.96;199.96;224.96;249.96;274.96;299.96;324.96;349.96;399.96;449.96;599.96], col_idx=[0 0.1 0.2 0.3 0.4 0.5 0.6 1]}
      mask prompts: table "Table Data"; row_idx "Breakpoints 1:"; col_idx "Breakpoints 2:"
      mask Display:
      | color('red');
      | fprintf('Prelookup\n2D');
      | 
      | color('black');
      | port_label('input', 1, 'u1');
      | port_label('input', 2, 'u2');
      | port_label('input', 3, 'u3');
      | port_label('input', 4, 'u4');
  SubSystem_12 : Subsystem  mask{table=[0 0.1 0.2 0.3 0.4 0.5 0.6 1;0 0.1 0.2 0.3 0.4 0.5 0.6 1;0 0.1 0.2 0.3 0.4 0.5 0.6 1;0 0.1 0.2 0.3 0.4 0.5 0.6 1;0 0.1 0.2 0.3 0.4 0.5 0.6 1;0 0.1 0.2 0.3 0.4 0.5 0.6 1;0 0.1 0.2 0.3 0.4 0.5 0.6 1;0 0.1 0.2 0.3 0.4 0.5 0.6 1;0 0.1 0.2 0.3 0.4 0.5 0.6 1;0 0.1 0.2 0.3 0.4 0.5 0.6 1;0 0.1 0.2 0.3 0.4 0.5 0.6 1;0 0.1 0.2 0.3 0.4 0.5 0.6 1], row_idx=[159.96;179.96;199.96;224.96;249.96;274.96;299.96;324.96;349.96;399.96;449.96;599.96], col_idx=[0 0.1 0.2 0.3 0.4 0.5 0.6 1]}
      mask prompts: table "Table Data"; row_idx "Breakpoints 1:"; col_idx "Breakpoints 2:"
      mask Display:
      | color('red');
      | fprintf('Prelookup\n2D');
      | 
      | color('black');
      | port_label('input', 1, 'u1');
      | port_label('input', 2, 'u2');
      | port_label('input', 3, 'u3');
      | port_label('input', 4, 'u4');
  SubSystem_3 : Subsystem  mask{table=[1 1 1 1 1 1 0.995 0.99 0.986 0.981 0.976 0.942;1 1 1 1 1 1 0.997 0.994 0.991 0.985 0.978 0.949;1 1 1 1 1 1 0.999 0.998 0.996 0.988 0.98 0.957;1 1 1 1 1 1 0.99 0.99 0.99 0.991 0.982 0.966;1 1 1 1 1 1 0.99 0.99 0.99 0.992 0.985 0.976;1 1 1 1 1 1 0.99 0.99 0.99 0.993 0.987 0.985;1 1 1 1 1 1 0.99 0.99 0.99 0.994 0.988 0.986;1 1 1 1 1 1 0.99 0.99 0.99 0.994 0.989 0.987;1 1 1 1 1 1 0.99 0.99 0.99 0.995 0.99 0.988;1 1 1 1 1 1 0.99 0.99 0.99 0.996 0.992 0.99;1 1 1 1 1 1 0.99 0.99 0.99 0.996 0.993 0.993;1 1 1 1 1 1 1 1 1 1 0.999 0.999], row_idx=[159.96;179.96;199.96;224.96;249.96;274.96;299.96;324.96;349.96;399.96;449.96;599.96], col_idx=[0 100 200 300 400 500 600 700 800 900 1000 1500]}
      mask prompts: table "Table Data"; row_idx "Breakpoints 1:"; col_idx "Breakpoints 2:"
      mask Display:
      | color('red');
      | fprintf('Prelookup\n2D');
      | 
      | color('black');
      | port_label('input', 1, 'u1');
      | port_label('input', 2, 'u2');
      | port_label('input', 3, 'u3');
      | port_label('input', 4, 'u4');
  SubSystem_4 : Subsystem  mask{table=[1 1 1 1 1 1 1 0.998 0.994 0.989 0.984 0.95;1 1 1 1 1 1 1 1 0.999 0.993 0.986 0.957;1 1 1 1 1 1 1 1 1 0.996 0.988 0.965;1 1 1 1 1 1 1 1 1 0.999 0.99 0.974;1 1 1 1 1 1 1 1 1 1 0.993 0.984;1 1 1 1 1 1 1 1 1 1 0.995 0.993;1 1 1 1 1 1 1 1 1 1 0.996 0.994;1 1 1 1 1 1 1 1 1 1 0.997 0.995;1 1 1 1 1 1 1 1 1 1 0.998 0.996;1 1 1 1 1 1 1 1 1 1 1 0.998;1 1 1 1 1 1 1 1 1 1 1 1;1 1 1 1 1 1 1 1 1 1 1 1], row_idx=[159.96;179.96;199.96;224.96;249.96;274.96;299.96;324.96;349.96;399.96;449.96;599.96], col_idx=[0 100 200 300 400 500 600 700 800 900 1000 1500]}
      mask prompts: table "Table Data"; row_idx "Breakpoints 1:"; col_idx "Breakpoints 2:"
      mask Display:
      | color('red');
      | fprintf('Prelookup\n2D');
      | 
      | color('black');
      | port_label('input', 1, 'u1');
      | port_label('input', 2, 'u2');
      | port_label('input', 3, 'u3');
      | port_label('input', 4, 'u4');
  SubSystem_5 : Subsystem  mask{table=[0.931 0.962 0.969 0.976 0.993 1 0.96 0.92 0.88 0.84 0.804 0.8;0.941 0.973 0.977 0.982 0.996 1 0.961 0.922 0.883 0.844 0.809 0.805;0.945 0.976 0.984 0.988 0.999 1 0.962 0.924 0.885 0.847 0.813 0.809;0.95 0.981 0.988 0.99 1 1 0.963 0.926 0.889 0.852 0.819 0.815;0.96 0.986 0.992 0.995 1 1 0.964 0.928 0.892 0.856 0.824 0.82;0.97 1 1 1 1 1 0.965 0.93 0.896 0.861 0.829 0.826;0.98 1 1 1 1 1 0.966 0.933 0.899 0.866 0.835 0.832;0.99 1 1 1 1 1 0.968 0.935 0.903 0.87 0.841 0.838;1 1 1 1 1 1 0.969 0.937 0.906 0.874 0.846 0.843;1 1 1 1 1 1 0.971 0.942 0.913 0.884 0.858 0.855;1 1 1 1 1 1 0.973 0.946 0.92 0.893 0.869 0.866;1 1 1 1 1 1 0.98 0.96 0.94 0.92 0.902 0.9], row_idx=[159.96;179.96;199.96;224.96;249.96;274.96;299.96;324.96;349.96;399.96;449.96;599.96], col_idx=[0 0.1 0.2 0.3 0.4 0.5 0.6 0.7 0.8 0.9 0.99 1]}
      mask prompts: table "Table Data"; row_idx "Breakpoints 1:"; col_idx "Breakpoints 2:"
      mask Display:
      | color('red');
      | fprintf('Prelookup\n2D');
      | 
      | color('black');
      | port_label('input', 1, 'u1');
      | port_label('input', 2, 'u2');
      | port_label('input', 3, 'u3');
      | port_label('input', 4, 'u4');
  SubSystem_6 : Subsystem  mask{table=[0.931 0.962 0.969 0.976 0.993 1 0.96 0.92 0.88 0.84 0.804 0.8;0.941 0.973 0.977 0.982 0.996 1 0.961 0.922 0.883 0.844 0.809 0.805;0.945 0.976 0.984 0.988 0.999 1 0.962 0.924 0.885 0.847 0.813 0.809;0.95 0.981 0.988 0.99 1 1 0.963 0.926 0.889 0.852 0.819 0.815;0.96 0.986 0.99 0.99 1 1 0.964 0.928 0.892 0.856 0.824 0.82;0.97 1 1 1 1 1 0.965 0.93 0.896 0.861 0.829 0.826;0.98 1 1 1 1 1 0.966 0.933 0.899 0.866 0.835 0.832;0.99 1 1 1 1 1 0.968 0.935 0.903 0.87 0.841 0.838;1 1 1 1 1 1 0.969 0.937 0.906 0.874 0.846 0.843;1 1 1 1 1 1 0.971 0.942 0.913 0.884 0.858 0.855;1 1 1 1 1 1 0.973 0.946 0.92 0.893 0.869 0.866;1 1 1 1 1 1 0.98 0.96 0.94 0.92 0.902 0.9], row_idx=[159.96;179.96;199.96;224.96;249.96;274.96;299.96;324.96;349.96;399.96;449.96;599.96], col_idx=[0 0.1 0.2 0.3 0.4 0.5 0.6 0.7 0.8 0.9 0.99 1]}
      mask prompts: table "Table Data"; row_idx "Breakpoints 1:"; col_idx "Breakpoints 2:"
      mask Display:
      | color('red');
      | fprintf('Prelookup\n2D');
      | 
      | color('black');
      | port_label('input', 1, 'u1');
      | port_label('input', 2, 'u2');
      | port_label('input', 3, 'u3');
      | port_label('input', 4, 'u4');
  SubSystem_7 : Subsystem  mask{table=[1 1 1 1 1 1 1 1 1 1 1 1;1 1 1 1 1 1 1 1 1 1 1 1;1 1 1 1 1 1 1 1 1 1 1 0.999;1 1 1 1 1 1 1 1 1 0.999 0.999 0.997;1 1 1 1 1 1 1 1 1 0.999 0.998 0.996;1 1 1 1 1 1 1 1 0.999 0.998 0.997 0.994;1 1 1 1 1 1 1 1 0.999 0.997 0.996 0.993;1 1 1 1 1 1 1 0.999 0.997 0.996 0.994 0.991;1 1 1 1 1 1 1 0.998 0.997 0.995 0.994 0.99;1 1 1 1 1 1 1 0.998 0.997 0.995 0.993 0.989;1 1 1 1 1 1 1 0.998 0.996 0.994 0.993 0.988;1 1 1 1 1 1 0.998 0.997 0.995 0.993 0.991 0.987], row_idx=[159.96;179.96;199.96;224.96;249.96;274.96;299.96;324.96;349.96;399.96;449.96;599.96], col_idx=[0 125 250 500 750 1000 1200 1400 1600 1800 2000 2500]}
      mask prompts: table "Table Data"; row_idx "Breakpoints 1:"; col_idx "Breakpoints 2:"
      mask Display:
      | color('red');
      | fprintf('Prelookup\n2D');
      | 
      | color('black');
      | port_label('input', 1, 'u1');
      | port_label('input', 2, 'u2');
      | port_label('input', 3, 'u3');
      | port_label('input', 4, 'u4');
  SubSystem_8 : Subsystem  mask{table=[0.268 0.285 0.296 0.309 0.337 0.407 0.541 0.629 0.786 0.96 0.96 0.96;0.316 0.333 0.343 0.356 0.384 0.452 0.583 0.669 0.819 0.97 0.97 0.97;0.366 0.382 0.392 0.405 0.432 0.498 0.626 0.709 0.851 0.981 0.981 0.981;0.429 0.445 0.454 0.466 0.492 0.556 0.678 0.758 0.89 0.992 0.992 0.992;0.491 0.506 0.515 0.526 0.551 0.611 0.724 0.8 0.92 0.998 0.998 0.998;0.55 0.564 0.572 0.583 0.606 0.661 0.766 0.835 0.939 0.998 0.998 0.998;0.604 0.617 0.625 0.635 0.657 0.71 0.81 0.871 0.954 0.996 0.996 0.996;0.655 0.668 0.676 0.686 0.708 0.76 0.856 0.909 0.969 0.996 0.996 0.996;0.7 0.714 0.722 0.733 0.755 0.809 0.907 0.95 0.986 0.996 0.996 0.996;0.757 0.774 0.785 0.798 0.824 0.892 0.993 0.993 0.993 0.993 0.993 0.993;0.775 0.789 0.797 0.807 0.827 0.881 0.981 0.988 0.988 0.988 0.988 0.988;0.763 0.852 0.856 0.859 0.868 0.891 0.933 0.97 0.97 0.97 0.97 0.97], row_idx=[159.96;179.96;199.96;224.96;249.96;274.96;299.96;324.96;349.96;399.96;449.96;599.96], col_idx=[0 0.24 0.38 0.55 0.92 1.85 3.66 4.81 7.39 9.62 24.05 34.2]}
      mask prompts: table "Table Data"; row_idx "Breakpoints 1:"; col_idx "Breakpoints 2:"
      mask Display:
      | color('red');
      | fprintf('Prelookup\n2D');
      | 
      | color('black');
      | port_label('input', 1, 'u1');
      | port_label('input', 2, 'u2');
      | port_label('input', 3, 'u3');
      | port_label('input', 4, 'u4');
  SubSystem_9 : Subsystem  mask{table=[0.279 0.297 0.308 0.322 0.351 0.424 0.564 0.655 0.819 1 1 1;0.326 0.343 0.354 0.367 0.396 0.466 0.601 0.69 0.844 1 1 1;0.373 0.389 0.4 0.413 0.44 0.508 0.638 0.723 0.868 1 1 1;0.432 0.448 0.458 0.47 0.496 0.56 0.683 0.764 0.897 1 1 1;0.492 0.507 0.516 0.527 0.552 0.612 0.726 0.802 0.922 1 1 1;0.551 0.565 0.573 0.584 0.607 0.662 0.768 0.837 0.941 1 1 1;0.607 0.62 0.628 0.638 0.66 0.713 0.813 0.875 0.958 1 1 1;0.658 0.671 0.679 0.689 0.711 0.763 0.86 0.913 0.973 1 1 1;0.703 0.717 0.725 0.736 0.758 0.813 0.911 0.954 0.99 1 1 1;0.762 0.779 0.79 0.803 0.83 0.898 1 1 1 1 1 1;0.784 0.798 0.806 0.816 0.837 0.891 0.992 1 1 1 1 1;0.78 0.878 0.882 0.886 0.895 0.918 0.962 1 1 1 1 1], row_idx=[159.96;179.96;199.96;224.96;249.96;274.96;299.96;324.96;349.96;399.96;449.96;599.96], col_idx=[0 0.24 0.38 0.55 0.92 1.85 3.66 4.81 7.39 9.62 24.05 34.2]}
      mask prompts: table "Table Data"; row_idx "Breakpoints 1:"; col_idx "Breakpoints 2:"
      mask Display:
      | color('red');
      | fprintf('Prelookup\n2D');
      | 
      | color('black');
      | port_label('input', 1, 'u1');
      | port_label('input', 2, 'u2');
      | port_label('input', 3, 'u3');
      | port_label('input', 4, 'u4');
  Switch2 : Switch  Criteria=u2 ~= 0  Threshold=SOUIT
  ATS_etaEstNOxCnvUCat : Outport
  wires:
  ATS_tEstUCatAvrg/1 -> PreLookup_7/1
  PreLookup_3/2 -> SubSystem_8/4(In4), SubSystem_9/4(In4)
  PreLookup_3/1 -> SubSystem_8/3(In3), SubSystem_9/3(In3)
  SubSystem_8/1(Out1) -> Mux1/1
  SubSystem_9/1(Out1) -> Mux1/2
  Mux1/1 -> Interpolation Using Prelookup/3
  SubSystem_12/1(Out1) -> Prelookup/1
  Interpolation Using Prelookup/1 -> Switch2/1  "SCRMod_etaTempNH3Ld_mp"
  ATS_facEffUCatAge/1 -> PreLookup_2/1
  PreLookup_1/2 -> SubSystem_4/4(In4), SubSystem_3/4(In4)
  PreLookup_1/1 -> SubSystem_4/3(In3), SubSystem_3/3(In3)
  SubSystem_3/1(Out1) -> Mux2/1
  SubSystem_4/1(Out1) -> Mux2/2
  Mux2/1 -> Interpolation Using Prelookup1/3
  PreLookup_2/1 -> SubSystem_12/3(In3), SubSystem_11/3(In3)
  PreLookup_2/2 -> SubSystem_12/4(In4), SubSystem_11/4(In4)
  SubSystem_11/1(Out1) -> Prelookup1/1
  Prelookup1/1 -> Interpolation Using Prelookup1/1, Interpolation Using Prelookup2/1
  Prelookup1/2 -> Interpolation Using Prelookup1/2, Interpolation Using Prelookup2/2
  Interpolation Using Prelookup1/1 -> Product1/2  "SCRMod_etaCorEG_mp"
  PreLookup_7/2 -> SubSystem_12/2(In2), SubSystem_8/2(In2), SubSystem_9/2(In2), SubSystem_10/2(In2), SubSystem_11/2(In2), SubSystem_3/2(In2), SubSystem_4/2(In2), SubSystem_5/2(In2), SubSystem_7/2(In2), SubSystem_6/2(In2)
  PreLookup_5/2 -> SubSystem_6/4(In4), SubSystem_5/4(In4)
  PreLookup_5/1 -> SubSystem_6/3(In3), SubSystem_5/3(In3)
  SubSystem_5/1(Out1) -> Mux3/1
  SubSystem_6/1(Out1) -> Mux3/2
  Mux3/1 -> Interpolation Using Prelookup2/3
  Prelookup/1 -> Interpolation Using Prelookup/1
  Prelookup/2 -> Interpolation Using Prelookup/2
  Interpolation Using Prelookup2/1 -> Product1/3  "SCRMod_etaCorNO2_mp"
  PreLookup_6/1 -> SubSystem_7/3(In3)
  PreLookup_6/2 -> SubSystem_7/4(In4)
  PreLookup_4/1 -> SubSystem_10/3(In3)
  PreLookup_4/2 -> SubSystem_10/4(In4)
  SubSystem_7/1(Out1) -> Product1/4  "SCRMod_etaCorNOxUs_mp"
  Constant/1 -> Product1/5  "SCRMod_facEstHCLd_mp"
  Switch2/1 -> Product1/1
  Divide2/1 -> PreLookup_4/1  "SCRMod_rEstNH3Ld"
  ATS_mflEG/1 -> PreLookup_1/1
  ATS_rNO2NOxUCatUs/1 -> PreLookup_5/1
  ATS_rNOxUCatUs_ppm/1 -> PreLookup_6/1
  SCRLdG_mNH3LdNom/1 -> Divide2/2
  PreLookup_7/1 -> SubSystem_12/1(In1), SubSystem_8/1(In1), SubSystem_9/1(In1), SubSystem_10/1(In1), SubSystem_11/1(In1), SubSystem_3/1(In1), SubSystem_4/1(In1), SubSystem_5/1(In1), SubSystem_7/1(In1), SubSystem_6/1(In1)
  SubSystem_10/1(Out1) -> Switch2/3
  Constant_1/1 -> Switch2/2
  Product1/1 -> Multiport Switch/2
  ATS_mflNH3Cnv_mgs/1 -> Relational Operator/1
  Constant3/1 -> Multiport Switch/3
  Constant2/1 -> Relational Operator1/2
  Logical Operator/1 -> Multiport Switch/1
  Relational Operator/1 -> Logical Operator/1
  Relational Operator1/1 -> Logical Operator/2
  Constant1/1 -> Relational Operator/2
  ATS_mEstNH3LdUCat/1 -> Relational Operator1/1, Divide2/1, PreLookup_3/1
  Multiport Switch/1 -> ATS_etaEstNOxCnvUCat/1
